simulink model "controller_stateflow"  (R2022b)
settings: Solver=FixedStepAuto  StartTime=0.0  StopTime=inf  FixedStep=0.05  RelTol=1e-3
PreLoadFcn:
  | rosinit();
model workspace (MAT data in the model file):
  SL_ROS_VariableLengthArrays_MaxSizes : object (value not decoded)
  pitch = -10
  restart = 0
values from neighbouring files (symbols this model uses):
  Pose = distance*inv(toPandatf)*Pose_d0    [inverseContoller3.m]    (also in inverseContoller4.m = distance*inv(toUR10etf)*Point_d0; inverseContoller_dual.m = inv(toUR10etf)*Point_d0; inverseContoller_dual2.m = inv(toUR10etf)*Point_d0)
undefined symbols (not defined in the file or in its folder): StartTime
libraries: robotmaniplib x25, robotlib x19, robotcorelib x3, robotgazebolib x1
(part 2 of 2)

== stateflow chart controller_stateflow/Chart3 ==
  state [ur_pos,durTime_ur] = get_ur_pose(box_pose,box_ZYX,sum_actual_pos,sum_actual_ZYX,ur_state,state) [function]
  state [ur_pos1,durTime_ur] = get_ur_pose_tra(tra_pos,tra_ZYX,sum_actual_pos,sum_actual_ZYX,ur_state,state) [function]
  state [panda_pos,durTime_panda] = get_panda_pose(box_pos,box_ZYX,sum_actual_pos,sum_actual_ZYX,panda_state,state) [function]
  state [panda_pos,durTime_panda] = get_panda_pose_track(box_pos,box_ZYX,sum_actual_pos,sum_actual_ZYX,panda_state,state) [function]
  state Initialization [group]
    state initial_state
      entry:
      fprintf("State flow started... \n");
      sum_pos = [0;0;0];
      sum_ZYX = [0;0;0];
      send_command_ur10e = 0;
      send_command_panda = 0;
      send_command_sum = 0;
      E_panda_track = 0;
      panda_durTime = 2;
      ur_durTime = 2;
      state_velvet = 0;
    state initial_pose
      entry: fprintf("Go to initial_pose \n");
      [ur_pos,ur_durTime] = set_ur_initialState(ur_state);
      [panda_pos,panda_durTime] = set_panda_initialState(panda_state);
      during:
      send_command_ur10e = 1;
      send_command_panda = 1;
      send_command_sum = 1;
    state Ready
      entry: fprintf("initial_pose done! \n");
      send_command_ur10e = 0;
      send_command_panda = 0;
      send_command_sum = 0;
    (default) -> initial_state
    initial_state -> initial_pose : [controller_ready && link_state_ready]
    initial_pose -> Ready : [ur_finish && panda_finish && sum_finish]
  state Release [group]
    state go_near_the_transporter
      entry:
      fprintf("go near the transporter ... \n");
      during:
      distance_from_tra = 0.7;
      distance_xx = 0.3;
      [sum_pos,sum_ZYX] = get_sum_pose_from_tra(tra_pos,tra_ZYX,distance_from_tra,distance_xx);
      send_command_sum = 1;
    state Set_initial_ee_poses
      entry: fprintf("set initial ee poses \n");
      send_command_ur10e = 0;
      send_command_panda = 0;
      send_command_sum = 0;
      E_panda_track = 1;
      [ur_pos,ur_durTime] = get_ur_pose_tra(tra_pos,tra_ZYX,sum_actual_pos,sum_actual_ZYX,ur_state,1);
      during:
      send_command_ur10e=1;
      [panda_pos, panda_durTime] = get_panda_pose_track(box_pos,box_ZYX,sum_actual_pos,sum_actual_ZYX,panda_state,122);
    state Go_near_the_transporter
      entry:
      fprintf("Going near near the transporter ... \n");
      send_command_ur10e = 0;
      send_command_panda = 0;
      E_panda_track = 0;
      panda_durTime = 2;
      ur_durTime = 2;
      during:
      [sum_pos,sum_ZYX] = get_sum_pose_from_tra(tra_pos,tra_ZYX,distance_from_tra,distance_xx-0.3);
      send_command_sum = 1;
    state ok
      entry: fprintf("ok.. \n ");
      send_command_ur10e = 0;
      send_command_panda = 0;
      send_command_sum = 0;
    state Pick_out1
      entry: fprintf("SofHand up \n");
      [panda_pos, panda_durTime] = get_panda_pose(box_pos,box_ZYX,sum_actual_pos,sum_actual_ZYX,panda_state,13);
      during:
      send_command_panda = 1;
    state Pick_out2
      entry: fprintf("Box Off \n");
      during:
      state_velvet = -1; %pick-off
    state ok1
      entry: fprintf("Success! \n ");
      send_command_ur10e = 0;
      send_command_panda = 0;
      send_command_sum = 0;
    state go_back_from_the_transporter
      entry:
      fprintf("Go back from the transporter ... \n");
      during:
      distance_from_tra = 0.8;
      distance_xx = 0.3;
      [sum_pos,sum_ZYX] = get_sum_pose_from_tra(tra_pos,tra_ZYX,distance_from_tra,distance_xx);
      send_command_sum = 1;
    go_near_the_transporter -> Release.Set_initial_ee_poses : [sum_finish && go>11]
    Release.Set_initial_ee_poses -> Go_near_the_transporter : [ur_finish  && go>12]
    Go_near_the_transporter -> Release.ok : [sum_finish && 1]
    Release.ok -> Pick_out1 : [go>13]
    Pick_out1 -> Pick_out2 : [panda_finish && go>14]
    Pick_out2 -> Release.ok1 : [box_off && go>15]{state_velvet = 0;}
    Release.ok1 -> go_back_from_the_transporter
  state Primitive_2 [group]
    state Go_to_Box
      entry:
      fprintf("go near the box ... \n");
      during:
      distance_from_box = 0.8;
      distance_10 = 0.35;
      [sum_pos,sum_ZYX] = get_sum_pose_from_box(box_pos,box_ZYX,distance_from_box,distance_10);
      send_command_sum = 1;
    state Set_initial_ee_poses
      entry: fprintf("set initial ee poses ");
      send_command_ur10e = 0;
      send_command_panda = 0;
      send_command_sum = 0;
      [ur_pos,ur_durTime] = get_ur_pose(box_pos,box_ZYX,sum_actual_pos,sum_actual_ZYX,ur_state,10);
      [panda_pos, panda_durTime] = get_panda_pose(box_pos,box_ZYX,sum_actual_pos,sum_actual_ZYX,panda_state,10);
      during:
      send_command_ur10e=1;
      send_command_panda = 1;
    state Go_near_the_box
      entry:
      fprintf("Going near the box ... \n");
      distance_10 = 0;
      during:
      [sum_pos,sum_ZYX] = get_sum_pose_from_box(box_pos,box_ZYX,distance_from_box,distance_10);
      send_command_sum = 1;
    state ok
      entry: fprintf("ok \n");
      send_command_ur10e = 0;
      send_command_panda = 0;
      send_command_sum = 0;
    state Pick_box1
      entry: fprintf("sofhand goes down \n");
      [panda_pos, panda_durTime]  = get_panda_pose(box_pos,box_ZYX,sum_actual_pos,sum_actual_ZYX,panda_state,11);
      during:
      send_command_panda = 1;
    state Pick_box2
      entry: fprintf("get box on velvet \n ");
      send_command_panda = 0;
      [panda_pos, panda_durTime]  = get_panda_pose(box_pos,box_ZYX,sum_actual_pos,sum_actual_ZYX,panda_state,12);
      during:
      send_command_panda = 1;
      state_velvet = 1; %pick-up
    state ok1
      entry: fprintf("success pick up box \n");
      send_command_ur10e = 0;
      send_command_panda = 0;
      send_command_sum = 0;
    state Pick_box3
      entry: fprintf("Hold it \n");
      send_command_panda = 0;
      [panda_pos, panda_durTime]  = get_panda_pose(box_pos,box_ZYX,sum_actual_pos,sum_actual_ZYX,panda_state,122);
      during:
      send_command_panda = 1;
    state ok2
      entry: fprintf("ok \n");
      send_command_ur10e = 0;
      send_command_panda = 0;
      send_command_sum = 0;
    state go_back_from_the_box
      entry:
      fprintf("go back from the box ... \n");
      distance_from_box = 0.8;
      distance_10 = 0.3;
      [sum_pos,sum_ZYX] = get_sum_pose_from_box(box_pos,box_ZYX,distance_from_box,distance_10);
      during:
      send_command_sum = 1;
    Primitive_2.Go_to_Box -> Primitive_2.Set_initial_ee_poses : [sum_finish && go>2]
    Primitive_2.Set_initial_ee_poses -> Primitive_2.Go_near_the_box : [ur_finish && panda_finish && go>3]
    Primitive_2.Go_near_the_box -> Primitive_2.ok : [sum_finish && go>4]
    Primitive_2.ok -> Primitive_2.Pick_box1 : [1 && go>5]
    Primitive_2.Pick_box1 -> Primitive_2.Pick_box2 : [panda_finish && go>6]
    Primitive_2.Pick_box2 -> Primitive_2.ok1 : [panda_finish && box_on_velvet]{state_velvet = 0;}
    Primitive_2.ok1 -> Primitive_2.Pick_box3 : [go>7]
    Primitive_2.Pick_box3 -> Primitive_2.ok2 : [panda_finish && go>8]
    Primitive_2.ok2 -> Primitive_2.go_back_from_the_box : [go>9]
  state Primitive_1 [group]
    state Go_to_Box
      entry:
      fprintf("go near the box ... \n");
      during:
      distance_from_box = 0.8;
      distance_10 = 0.3;
      [sum_pos,sum_ZYX] = get_sum_pose_from_box(box_pos,box_ZYX,distance_from_box,distance_10);
      send_command_sum = 1;
    state Set_initial_ee_poses
      entry: fprintf("set initial ee poses ");
      send_command_ur10e = 0;
      send_command_panda = 0;
      send_command_sum = 0;
      [ur_pos,ur_durTime] = get_ur_pose(box_pos,box_ZYX,sum_actual_pos,sum_actual_ZYX,ur_state,10);
      [panda_pos, panda_durTime] = get_panda_pose(box_pos,box_ZYX,sum_actual_pos,sum_actual_ZYX,panda_state,10);
      during:
      send_command_ur10e=1;
      send_command_panda = 1;
    state Go_near_the_box
      entry:
      fprintf("Going near the box ... \n");
      during:
      [sum_pos,sum_ZYX] = get_sum_pose_from_box(box_pos,box_ZYX,distance_from_box,distance_10-0.3);
      send_command_sum = 1;
    state ok
      entry: fprintf("ok \n");
      send_command_ur10e = 0;
      send_command_panda = 0;
      send_command_sum = 0;
    state Pick_box1
      entry: fprintf("sofhand goes down \n");
      [panda_pos, panda_durTime]  = get_panda_pose(box_pos,box_ZYX,sum_actual_pos,sum_actual_ZYX,panda_state,11);
      during:
      send_command_panda = 1;
    state Pick_box2
      entry: fprintf("get box on velvet \n ");
      send_command_panda = 0;
      [panda_pos, panda_durTime]  = get_panda_pose(box_pos,box_ZYX,sum_actual_pos,sum_actual_ZYX,panda_state,12);
      during:
      send_command_panda = 1;
      state_velvet = 1; %pick-up
    state ok1
      entry: fprintf("success pick up box \n");
      send_command_ur10e = 0;
      send_command_panda = 0;
      send_command_sum = 0;
    state Pick_box3
      entry: fprintf("Hold it \n");
      send_command_panda = 0;
      [panda_pos, panda_durTime]  = get_panda_pose(box_pos,box_ZYX,sum_actual_pos,sum_actual_ZYX,panda_state,122);
      during:
      send_command_panda = 1;
    state ok2
      entry: fprintf("ok \n");
      send_command_ur10e = 0;
      send_command_panda = 0;
      send_command_sum = 0;
    state go_back_from_the_box
      entry:
      fprintf("go back from the box ... \n");
      distance_from_box = 0.8;
      distance_10 = 0.3;
      [sum_pos,sum_ZYX] = get_sum_pose_from_box(box_pos,box_ZYX,distance_from_box,distance_10);
      during:
      send_command_sum = 1;
    Primitive_1.Go_to_Box -> Primitive_1.Set_initial_ee_poses : [sum_finish && go>2]
    Primitive_1.Set_initial_ee_poses -> Primitive_1.Go_near_the_box : [ur_finish && panda_finish && go>3]
    Primitive_1.Go_near_the_box -> Primitive_1.ok : [sum_finish && go>4]
    Primitive_1.ok -> Primitive_1.Pick_box1 : [1 && go>5]
    Primitive_1.Pick_box1 -> Primitive_1.Pick_box2 : [panda_finish && go>6]
    Primitive_1.Pick_box2 -> Primitive_1.ok1 : [panda_finish && box_on_velvet && go>7]{state_velvet = 0;}
    Primitive_1.ok1 -> Primitive_1.Pick_box3
    Primitive_1.Pick_box3 -> Primitive_1.ok2 : [panda_finish && go>8]
    Primitive_1.ok2 -> Primitive_1.go_back_from_the_box : [go>9]
  state Finish [group]
    state Return_home
      entry:
      send_command_sum = 0;
      fprintf(" Return to home position ... \n");
      during:
      sum_pos = [0;0;0];
      sum_ZYX = [0;0;0];
      [ur_pos,ur_durTime] = set_ur_initialState(ur_state);
      [panda_pos,panda_durTime] = set_panda_initialState(panda_state);
      send_command_ur10e = 1;
      send_command_panda = 1;
      send_command_sum = 1;
    state finish
      entry: fprintf(" Mission Completed ! \n");
      send_command_ur10e = 0;
      send_command_panda = 0;
      send_command_sum = 0;
    Return_home -> Finish.finish : [ur_finish && panda_finish && sum_finish]
  state THE_END
  state Return home with box [group]
    state Go_back
      entry:
      send_command_sum = 0;
      fprintf("back ... \n ");
      during:
      sum_pos = [0;0;0];
      sum_ZYX = [0;0;0];
      send_command_sum = 1;
    state finish
      entry: fprintf("Home position reached...\n");
      send_command_ur10e = 0;
      send_command_panda = 0;
      send_command_sum = 0;
    Go_back -> Return.finish : [sum_finish]
  Return.finish -> go_near_the_transporter : [go>11]
  Ready -> Primitive_2.Go_to_Box [order 2] : [pick_type == 2 && go>1]
  Ready -> Primitive_1.Go_to_Box [order 1] : [pick_type == 1 && go>1]
  go_back_from_the_transporter -> Return_home : [sum_finish && go>16]
  Finish.finish -> THE_END
  Primitive_2.go_back_from_the_box -> Go_back : [sum_finish && go>10]
  Primitive_1.go_back_from_the_box -> Go_back : [sum_finish && go>10]
  data: ur_stat function_input; ur_Pos function_output; ur_durTime_ function_output; panda_pos function_output; panda_durTime_ function_output; panda_stat function_input; sum_pos function_output; sum_ZYX function_output; box_pos function_input; box_ZYX function_input; distance_from_box function_input; distance_10 function_input; sum_pos function_output; sum_ZYX function_output; tra_pos function_input; tra_ZYX function_input; distance_from_tra function_input; distance_xx function_input; box_pose function_input double size=[3,1]; box_ZYX function_input double size=[3,1]; sum_actual_pos function_input double size=[3,1]; sum_actual_ZYX function_input double size=[3,1]; ur_state function_input double size=[7,1]; ur_pos function_output; state function_input double size=1; durTime_ur function_output; tra_pos function_input double size=[3,1]; tra_ZYX function_input double size=[3,1]; sum_actual_pos function_input double size=[3,1]; sum_actual_ZYX function_input double size=[3,1]; ur_state function_input double size=[7,1]; state function_input double size=1; ur_pos1 function_output; durTime_ur function_output; box_pos function_input double size=[3,1]; box_ZYX function_input double size=[3,1]; sum_actual_pos function_input double size=[3,1]; sum_actual_ZYX function_input double size=[3,1]; panda_state function_input double size=[7,1]; panda_pos function_output; state function_input double size=1; durTime_panda function_output; box_pos function_input double size=[3,1]; box_ZYX function_input double size=[3,1]; sum_actual_pos function_input double size=[3,1]; sum_actual_ZYX function_input double size=[3,1]; panda_state function_input double size=[7,1]; panda_pos function_output; state function_input double size=1; durTime_panda function_output; sf_internal_action_state_placeholder_data local double size=1 =0; send_command_ur10e output size=1,1; controller_ready input; link_state_ready input; send_command_panda output; send_command_sum output; ur_pos output; ur_durTime output; panda_pos output; sum_pos output; panda_state input; ur_state input; panda_finish input; sum_finish input; ur_finish input; go input; box_ZYX input; sum_ZYX output; box_pos input; sum_actual_ZYX input; sum_actual_pos input; distance_10 local; distance_from_box local; box_on_velvet input; tra_ZYX input; tra_pos input; distance_from_tra local; distance_xx local; state_velvet output; E_panda_track output; panda_durTime output; box_off input; pick_type input
  function [ur_Pos,ur_durTime_]= set_ur_initialState(ur_stat):
    | function [ur_Pos,ur_durTime_]= set_ur_initialState(ur_stat)
    |  ur_pos_ = [       -0.6416   -5.6222+2*pi   -2.4013   -4.5429+2*pi    0.9292   -3.1416]';
    |     ur_pos_ = [-0.5247    1.2071   -2.5137    6.0191-2*pi   -4.7124+2*pi   -2.6169]';
    |   ur_Pos = horzcat(ur_pos_,ur_pos_,ur_pos_,ur_pos_,ur_pos_);
    | 
    |  ur_durTime_ = 3;
    | end
  function [panda_pos,panda_durTime_] = set_panda_initialState(panda_stat):
    | function [panda_pos,panda_durTime_] = set_panda_initialState(panda_stat)
    |  panda_pos_ = [0;-0.7853;0;-2.35619;0;1.57079;0.785398];
    |  panda_pos = horzcat(panda_pos_,panda_pos_,panda_pos_,panda_pos_,panda_pos_);
    |  panda_durTime_ = 3;
    | end
  function [sum_pos,sum_ZYX] = get_sum_pose_from_box(box_pos,box_ZYX,distance_from_box,distance_10):
    | function [sum_pos,sum_ZYX] = get_sum_pose_from_box(box_pos,box_ZYX,distance_from_box,distance_10)
    |     
    |     base_sum_length = 0.75; 
    |     
    |     % questo mi calcola la posizione in cui deve andare il robot, partendo
    |     % dalla posizione del box e aggiungendo un vettore distanza verso
    |     % l'asse y negativo del box
    |     back_from_box = box_pos + [eul2rotm(box_ZYX', 'ZYX')]*[0; -distance_from_box - distance_10 - base_sum_length/2;0];
    |     
    |     sum_pos = [back_from_box(1);back_from_box(2);0];
    | 
    |     % l'orientazione è solo relativa alla posa della scatola sul piano XY
    |     % ed è solo ruotata di 90 gradi
    |     sum_ZYX = [box_ZYX(1)+pi/2;0;0];  
    | 
    | end
  function [sum_pos,sum_ZYX] = get_sum_pose_from_tra(tra_pos,tra_ZYX,distance_from_tra,distance_xx):
    | function [sum_pos,sum_ZYX] = get_sum_pose_from_tra(tra_pos,tra_ZYX,distance_from_tra,distance_xx)
    |     
    |     base_sum_length = 0.75; 
    |         
    |     traDim = [1;5.456930;0.192575];
    | 
    |     back_from_box = tra_pos + [eul2rotm(tra_ZYX', 'ZYX')]*[0; traDim(2)/2 + +0.7+distance_xx + base_sum_length/2;0];
    |     
    |     sum_pos = [back_from_box(1);back_from_box(2);0];
    |     sum_ZYX = [tra_ZYX(1)-pi/2;0;0];  
    | 
    |         
    | end

== matlab function controller_stateflow/Subsystem6/MATLAB Function10 ==
  data: pos output; x input; quat output double; y input; z input; or_x input; or_y input; or_z input; or_w input
function [pos, quat] = fcn(x,y,z,or_x,or_y,or_z,or_w)
    
    pos=[x;y;z];
    quat=[or_w;or_x;or_y;or_z];

end

== matlab function controller_stateflow/MATLAB Function1 ==
  data: u input; y output double
function y = fcn(u)
y=0;
if u.Nsec > 1e8
y=1;
end

== matlab function controller_stateflow/MATLAB Function14 ==
  data: enable output; msgOut output Bus: SL_Bus_controller_stateflow_SetModelStateRequest_4q9jrn; msgIn input Bus: SL_Bus_controller_stateflow_SetModelStateRequest_4q9jrn; state input; boxPose input Bus: SL_Bus_controller_stateflow_geometry_msgs_Pose
function [enable,msgOut]  = fcn(msgIn,state,boxPose)

    msgOut = msgIn;
    
    bodyname = 'box_38_18_14';
    enable = 1;
    
    
    lenName = uint32(length(bodyname));
    msgOut.ModelState.ModelName(1:lenName,1) = uint8(convertStringsToChars(bodyname))';
    msgOut.ModelState.ModelName_SL_Info.CurrentLength = uint32(lenName);
   
    msgOut.ModelState.Pose = boxPose;

%     msgOut.ModelState.Twist.Linear.X=1.;
    
    msgOut.ModelState.Pose.Position.X = msgOut.ModelState.Pose.Position.X +0.02;


end
 

 
 
% enable = 0;
% y=0;
% 
% bodyname = 'box_38_18_14::link_0';
% lenName = uint32(length(bodyname));
% msgOut.BodyName_SL_Info.CurrentLength = uint32(lenName);
% msgOut.BodyName(1:lenName,1) = uint8(convertStringsToChars(bodyname))';
% 
% refname = 'iliad::ur10e_wrist_3_link';
% lenName = uint32(length(refname));
% msgOut.ReferenceFrame(1:lenName,1) = uint8(convertStringsToChars(refname))';
% msgOut.ReferenceFrame_SL_Info.CurrentLength = uint32(lenName);
% 
% msgOut.Wrench.Force.Y = 0;
% 
% if state == 12 && coll == 1
%     msgOut.Wrench.Force.Y = 0;
% 
%     msgOut.Wrench.Force.Z = -380;
% 
%     y=-0.0;
% end

== matlab function controller_stateflow/MATLAB Function2 ==
  data: u input; y output double
function y = fcn(u)
y=0;
if u.Sec >= 1
y=1;
end

== matlab function controller_stateflow/Chart3/get_panda_pose_track/MATLAB Function ==
  data: Pose output; boxPos input; boxZYX input; sumPos input; sumZYX input; panda_state input; Weights output; initialGuess output; state input; NWayPoints output; durTime output
function [Pose, Weights, initialGuess, NWayPoints, durTime] = fcn(boxPos,boxZYX,sumPos,sumZYX,panda_state,state)

    dimBox_x=0.38;
    dimBox_y=0.18;
    dimBox_z=0.14;
    
    toSumChapa = [0;0;0.51];
    toFranka = [0.25;-0.22;0.15];
    
    boxPos_offset = [0;0;0];
    
    boxtf_01 = [[eul2rotm(boxZYX', 'ZYX')],boxPos; ...
                0 0 0                               1           ];
    
    NWayPoints = 1;
    durTime = 2;
    
    if state == 122
        boxPos_offset = [0;+dimBox_y/2-0.05;dimBox_z/2+0.015];
        NWayPoints = 1;
        durTime = 0.3;
    end
    
    
    
    % boxPos0 = boxPos+boxPos_offset;
    
    boxPos0 = boxtf_01*[boxPos_offset;1];
    
    sumtf_01 = [[eul2rotm(sumZYX', 'ZYX')],sumPos; ...
                0 0 0                               1           ];
    sumtopandatf_12 = [[eul2rotm([0,pi/4,0], 'ZYX')],toSumChapa+toFranka; ...
                0 0 0                               1           ];
    
    toPandatf = sumtf_01*sumtopandatf_12;
    
    boxx = inv(toPandatf)*[boxPos0(1:3);1];
    
    
    Pose = [[eul2rotm([pi,0,0], 'ZYX')],[boxx(1);boxx(2);boxx(3)]; ...
                0 0 0                               1           ];
    
    if state == 122
        Pose = [[eul2rotm([pi,pi/8,0], 'ZYX')],[boxx(1);boxx(2);boxx(3)]; ...
                0 0 0                               1           ];
    end
    
    Weights = [1,1,1,1,1,1];
    initialGuess = panda_state;

end

== matlab function controller_stateflow/MATLAB Function12 ==
  data: enable output; msgOut output Bus: SL_Bus_controller_stateflow_ApplyBodyWrenchRequest_gxwnto; msgIn input Bus: SL_Bus_controller_stateflow_ApplyBodyWrenchRequest_gxwnto; state input; coll input; T_ur_velvCnt input
function [enable,msgOut]  = fcn(msgIn,state,coll,T_ur_velvCnt)

    msgOut = msgIn;
    
    bodyname = 'box_38_18_14::link_0';
    enable = 0;
    
    lenName = uint32(length(bodyname));
    msgOut.BodyName(1:lenName,1) = uint8(convertStringsToChars(bodyname))';
    msgOut.BodyName_SL_Info.CurrentLength = uint32(lenName);
   
    msgOut.ReferenceFrame(1:lenName,1) = uint8(convertStringsToChars(bodyname))';
    msgOut.ReferenceFrame_SL_Info.CurrentLength = uint32(lenName);
    
    msgOut.Wrench.Force.X =  0;
    msgOut.Wrench.Force.Y =  0;
    msgOut.Wrench.Force.Z =  0;
    msgOut.Wrench.Torque.X = 0;
    msgOut.Wrench.Torque.Y = 0;
    msgOut.Wrench.Torque.Z = 0;
        
    F_v = [0;0;0;1];

    if state == 1 && coll == 1
        k=0.75;
%         F_v = [0;0;-80*k;1];
        F_v = [-80*k;0;0;1];

        msgOut.Wrench.Torque.X = 0;
        msgOut.Wrench.Torque.Y = 0;
        msgOut.Wrench.Torque.Z = 0;

        msgOut.ReferencePoint.X = 0;
        msgOut.ReferencePoint.Y = 0;
        msgOut.ReferencePoint.Z = 0;
        
        msgOut.Duration.Sec = 0;
        msgOut.Duration.Nsec = 1e7;

        fprintf("pull \n");

        enable = 1;
    end


    if state == -1
        k=1.0;
%         F_v = [0;0;80*k;1];
        F_v = [80*k;0;0;1];

        msgOut.Wrench.Torque.X = 0;
        msgOut.Wrench.Torque.Y = 0;
        msgOut.Wrench.Torque.Z = 0;
        
        msgOut.ReferencePoint.X = 0;
        msgOut.ReferencePoint.Y = 0;
        msgOut.ReferencePoint.Z = 0;

        msgOut.Duration.Sec = 0;
        msgOut.Duration.Nsec = 1e7;

        fprintf("push \n");

        enable = 1;        
    end
        
    F_w = T_ur_velvCnt*F_v;

    msgOut.Wrench.Force.X = F_w(1);
    msgOut.Wrench.Force.Y = F_w(2);
    msgOut.Wrench.Force.Z = F_w(3);

end

== matlab function controller_stateflow/Subsystem/MATLAB Function1 ==
  data: Time input; msgOut output Bus: SL_Bus_controller_stateflow_trajectory_msgs_JointTrajectory; msgIn input; msgPoint input; TimeFromStart input; Point_array input
function msgOut   = fcn(Time, msgIn, msgPoint,TimeFromStart, Point_array)

    msgOut = msgIn;
    if Time.Sec ~= 0

        jointNames = {'ur10e_shoulder_pan_joint','ur10e_shoulder_lift_joint','ur10e_elbow_joint'...
            'ur10e_wrist_1_joint','ur10e_wrist_2_joint','ur10e_wrist_3_joint'};
        numJoints = uint32(length(jointNames));
        msgOut.JointNames_SL_Info.CurrentLength = numJoints;
        for idx = 1:numJoints
            jName = jointNames{idx};
            lenName = uint32(length(jName));
            msgOut.JointNames(idx).Data(1:lenName) = uint8(jName);
            msgOut.JointNames(idx).Data_SL_Info.CurrentLength = lenName;
        end

        msgOut.Header.Stamp.Sec = Time.Sec;
        msgOut.Header.Stamp.Nsec = Time.Nsec;
        
        msgOut.Header.Seq = uint32(0);

        if isequal(Point_array(:,1),Point_array(:,2))
            msgOut.Points_SL_Info.CurrentLength = uint32(1);
            msgOut.Points(1) = msgPoint;
            msgOut.Points(1).Positions(1:6) = Point_array(1:6,1);
            msgOut.Points(1).Positions_SL_Info.CurrentLength = uint32(6);
            msgOut.Points(1).TimeFromStart.Sec = TimeFromStart;
            msgOut.Points(1).TimeFromStart.Nsec = 0;
        else

            msgOut.Points_SL_Info.CurrentLength = uint32(size(Point_array,2));
    
            for i = 1:size(Point_array,2)
                msgOut.Points(i) = msgPoint;
                msgOut.Points(i).Positions(1:6) = Point_array(1:6,i);
                msgOut.Points(i).Positions_SL_Info.CurrentLength = uint32(6);
        
    %             msgOut.Points[i].Velocities(1:6) = [0 ;0 ;0 ;0 ;0 ;0];
    %             msgOut.Points[i].Velocities_SL_Info.CurrentLength = uint32(6);
    %             
    %             msgOut.Points[i].Accelerations(1:6) = [0 ;0 ;0 ;0 ;0 ;0];
    %             msgOut.Points[i].Accelerations_SL_Info.CurrentLength = uint32(6);
    %             
    %             msgOut.Points[i].Effort(1:6) = [0 ;0 ;0 ;0 ;0 ;0];
    %             msgOut.Points[i].Effort_SL_Info.CurrentLength = uint32(6);

                msgOut.Points(i).TimeFromStart.Sec = TimeFromStart + 1*i;
                msgOut.Points(i).TimeFromStart.Nsec = 0;
            end
        end
        
    end
end

== matlab function controller_stateflow/Chart3/get_ur_pose_tra/MATLAB Function ==
  data: Pose output; traPos input; traZYX input; sumPos input; sumZYX input; urState input; Weights output; initialGuess output; state input; NWayPoints output; durTime output
function [Pose, Weights, initialGuess ,NWayPoints,durTime] = fcn(traPos,traZYX,sumPos,sumZYX,urState,state)

traDim = [1;5.456930;0.192575];

% back_from_box = traPos + [eul2rotm(tra_ZYX', 'ZYX')]*[0; traDim(2)/2 + +0.7+distance_xx + base_sum_length/2;0];

toSumChapa = [0;0;0.51];
toUR10e = [0.35;0.32+0.02;0.05];

traPos_offset = [0;0;0];

velvet_length = 0.28+0.04;
velvet_height = 0.08;

base_ur_offset = [0;0;0.05];
NWayPoints = 1;
durTime = 2;

if state == 1
    traPos_offset = [eul2rotm(traZYX', 'ZYX')]*[0; traDim(2)/2 + velvet_length+0.3;-velvet_height/2+traDim(3)/2];
    NWayPoints = 1;
    durTime = 2;
end
if state == 2
    traPos_offset = [eul2rotm(traZYX', 'ZYX')]*[0; traDim(2)/2 + velvet_length;-velvet_height/2+traDim(3)/2+0.1];
    NWayPoints = 1;
    durTime = 2;
end


traPos0 = traPos+traPos_offset;

sumtf_01 = [[eul2rotm(sumZYX', 'ZYX')],sumPos; ...
            0 0 0                               1           ];
sumtoUR10etf_12 = [[eul2rotm([0,0,0], 'ZYX')],toSumChapa+toUR10e+base_ur_offset; ...
            0 0 0                               1           ];

toUR10etf = sumtf_01*sumtoUR10etf_12;


tra_ = inv(toUR10etf)*[traPos0;1];

Pose = [[eul2rotm([0,0,0], 'ZYX')],[tra_(1);tra_(2);tra_(3)]; ...
            0 0 0                               1           ];


Weights = [1,1,1,1,1,1];
initialGuess = urState(1:6,1);

end

== matlab function controller_stateflow/Subsystem5/MATLAB Function4 ==
  data: x output; T input; y output; box input; z output; sumPos input; sumZYX input; T_ur_velvCnt output; coll output; boxx output
function [x,y,z,T_ur_velvCnt,coll,boxx] = fcn(T,box,sumPos,sumZYX)
    
    dimBox = [0.38;0.18;0.14];
    
    toSumChapa = [0;0;0.51];
    toUR10e = [0.35;0.32;0.05];
    
    velvet_length = 0.28+0.04;
    velvet_height = 0.08;
    
    base_ur_offset = [0;0;0.05];
    
    sumtf_01 = [[eul2rotm(sumZYX', 'ZYX')],sumPos; ...
                0 0 0                               1           ];
    sumtoUR10etf_12 = [[eul2rotm([0,0,0], 'ZYX')],toSumChapa+toUR10e+base_ur_offset; ...
                0 0 0                               1           ];
    
    toUR10etf = sumtf_01*sumtoUR10etf_12;
    
    % with 'tool0' link transformation
%     to_velvCnt = [[eul2rotm([0,0,0], 'ZYX')],[0;-velvet_height/2-dimBox(3)/2;velvet_length-dimBox(2)/2]; ...
%                 0 0 0                               1           ];
    % with 'ee_link' link transformation
               to_velvCnt = [[eul2rotm([0,0,0], 'ZYX')],[velvet_length-dimBox(2)/2;0;velvet_height/2+dimBox(3)/2]; ...
     0 0 0                               1           ];
    
    T_ur_velvCnt = toUR10etf*T*to_velvCnt;
    
    boxx = inv(T_ur_velvCnt)*[box;1];
    
    x = boxx(1);
    y = boxx(2);
    z = boxx(3);
    
    coll = 0;
    
    goal = [0.165;0;0];
    tol = [0;0.05;0.05];
    
    if boxx(1) <= goal(1) - tol(1) && ...
       boxx(2) <= goal(2) + tol(2) && boxx(2) >= goal(2) - tol(2) && ...
       boxx(3) <= goal(3) + tol(3) && boxx(3) >= goal(3) - tol(3)
            coll = 1;
    end



end

== matlab function controller_stateflow/Subsystem5/MATLAB Function6 ==
  data: u input; y output
function y = fcn(u)

y = u(1:6);

== matlab function controller_stateflow/Subsystem5/MATLAB Function7 ==
  data: box_ok output; x input; y input; z input; tol input; box_off output
function [box_ok,box_off]  = fcn(x,y,z,tol)


    dimBox_x=0.38;
    dimBox_y=0.18;
    dimBox_z=0.14;
    velvet_length = 0.28+0.04;
    goal =[0,0,0];

    box_ok = 0;

    box_off = 0;

    if  x <= -0.01

        box_ok=1;

    end

    if  x >= 0.17

        box_off=1;

    end


end

== matlab function controller_stateflow/Chart3/get_ur_pose/MATLAB Function4 ==
  data: pose_d input; Pose1 output; T input; Pose2 output; Pose3 output; NWayPoint input; Pose4 output; Pose5 output
function [Pose1,Pose2,Pose3,Pose4,Pose5] = fcn(pose_d,T,NWayPoint)

    if NWayPoint == 1
        Pose1 = pose_d;
        Pose2 = pose_d;
        Pose3 = pose_d;
        Pose4 = pose_d;
        Pose5 = pose_d;
    else

        %semplice interpolazione lineare sulla posizione tra posizione
        %attuale e posizione desiderata
        pos_act   = T(1:3,4);
        pos_d     = pose_d(1:3,4);
        delta_pos = (pos_d-pos_act)/5; 

        Pose1 = [[eul2rotm([0,0,0], 'ZYX')],pos_act+delta_pos*1; ...
                 0 0 0                               1           ];
        Pose2 = [[eul2rotm([0,0,0], 'ZYX')],pos_act+delta_pos*2; ...
                 0 0 0                               1           ];
        Pose3 = [[eul2rotm([0,0,0], 'ZYX')],pos_act+delta_pos*3; ...
                 0 0 0                               1           ];
        Pose4 = [[eul2rotm([0,0,0], 'ZYX')],pos_act+delta_pos*4; ...
                 0 0 0                               1           ];

        Pose5 = pose_d;
    end

end

== matlab function controller_stateflow/Chart3/get_ur_pose/MATLAB Function6 ==
  data: u input; y output
function y = fcn(u)

y = u(1:6);

== matlab function controller_stateflow/Chart3/get_panda_pose_track/MATLAB Function4 ==
  data: pose_d input; Pose1 output; T input; Pose2 output; Pose3 output; NWayPoint input; Pose4 output; Pose5 output
function [Pose1,Pose2,Pose3,Pose4,Pose5] = fcn(pose_d,T,NWayPoint)

    if NWayPoint == 1
        Pose1 = pose_d;
        Pose2 = pose_d;
        Pose3 = pose_d;
        Pose4 = pose_d;
        Pose5 = pose_d;
    else

        %semplice interpolazione lineare sulla posizione tra posizione
        %attuale e posizione desiderata
        pos_act   = T(1:3,4);
        pos_d     = pose_d(1:3,4);
        delta_pos = (pos_d-pos_act)/5; 

        Pose1 = [[eul2rotm([0,0,0], 'ZYX')],pos_act+delta_pos*1; ...
                 0 0 0                               1           ];
        Pose2 = [[eul2rotm([0,0,0], 'ZYX')],pos_act+delta_pos*2; ...
                 0 0 0                               1           ];
        Pose3 = [[eul2rotm([0,0,0], 'ZYX')],pos_act+delta_pos*3; ...
                 0 0 0                               1           ];
        Pose4 = [[eul2rotm([0,0,0], 'ZYX')],pos_act+delta_pos*4; ...
                 0 0 0                               1           ];

        Pose5 = pose_d;
    end

end

== matlab function controller_stateflow/Chart3/get_ur_pose_tra/MATLAB Function4 ==
  data: pose_d input; Pose1 output; T input; Pose2 output; Pose3 output; NWayPoint input; Pose4 output; Pose5 output
function [Pose1,Pose2,Pose3,Pose4,Pose5] = fcn(pose_d,T,NWayPoint)

    if NWayPoint == 1
        Pose1 = pose_d;
        Pose2 = pose_d;
        Pose3 = pose_d;
        Pose4 = pose_d;
        Pose5 = pose_d;
    else

        %semplice interpolazione lineare sulla posizione tra posizione
        %attuale e posizione desiderata
        pos_act   = T(1:3,4);
        pos_d     = pose_d(1:3,4);
        delta_pos = (pos_d-pos_act)/5; 

        Pose1 = [[eul2rotm([0,0,0], 'ZYX')],pos_act+delta_pos*1; ...
                 0 0 0                               1           ];
        Pose2 = [[eul2rotm([0,0,0], 'ZYX')],pos_act+delta_pos*2; ...
                 0 0 0                               1           ];
        Pose3 = [[eul2rotm([0,0,0], 'ZYX')],pos_act+delta_pos*3; ...
                 0 0 0                               1           ];
        Pose4 = [[eul2rotm([0,0,0], 'ZYX')],pos_act+delta_pos*4; ...
                 0 0 0                               1           ];

        Pose5 = pose_d;
    end

end

== matlab function controller_stateflow/Chart3/get_ur_pose_tra/MATLAB Function6 ==
  data: u input; y output
function y = fcn(u)

y = u(1:6);

== matlab function controller_stateflow/Chart3/get_panda_pose/MATLAB Function4 ==
  data: pose_d input; Pose1 output; T input; Pose2 output; Pose3 output; NWayPoint input; Pose4 output; Pose5 output
function [Pose1,Pose2,Pose3,Pose4,Pose5] = fcn(pose_d,T,NWayPoint)

    if NWayPoint == 1
        Pose1 = pose_d;
        Pose2 = pose_d;
        Pose3 = pose_d;
        Pose4 = pose_d;
        Pose5 = pose_d;
    else

        %semplice interpolazione lineare sulla posizione tra posizione
        %attuale e posizione desiderata
        pos_act   = T(1:3,4);
        pos_d     = pose_d(1:3,4);
        delta_pos = (pos_d-pos_act)/5; 

        Pose1 = [[eul2rotm([0,0,0], 'ZYX')],pos_act+delta_pos*1; ...
                 0 0 0                               1           ];
        Pose2 = [[eul2rotm([0,0,0], 'ZYX')],pos_act+delta_pos*2; ...
                 0 0 0                               1           ];
        Pose3 = [[eul2rotm([0,0,0], 'ZYX')],pos_act+delta_pos*3; ...
                 0 0 0                               1           ];
        Pose4 = [[eul2rotm([0,0,0], 'ZYX')],pos_act+delta_pos*4; ...
                 0 0 0                               1           ];

        Pose5 = pose_d;
    end

end

== matlab function controller_stateflow/Chart3/get_panda_pose/MATLAB Function6 ==
  data: u input; y output
function y = fcn(u)

y = u(1:7);

== matlab function controller_stateflow/Chart3/get_panda_pose_track/MATLAB Function6 ==
  data: u input; y output
function y = fcn(u)

y = u(1:7);
